simulink library "LookupModeling"  (Simulink 7.7)
settings: Solver=ode45  StartTime=0.0  StopTime=10.0  RelTol=1e-3
settings Model: Creator=medcps  LastModifiedBy=iris

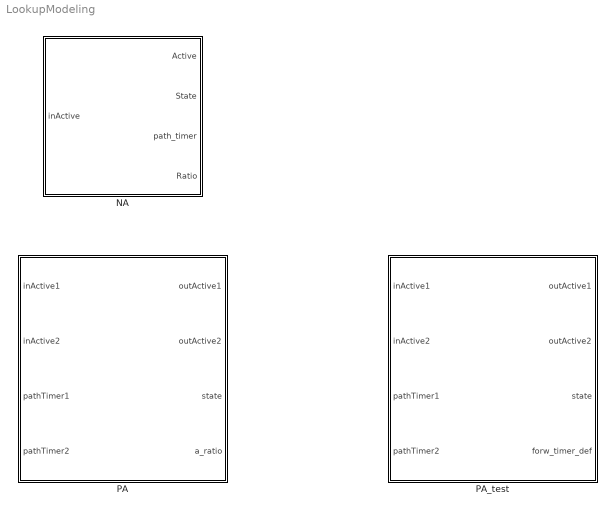
== system LookupModeling ==
  NA : Subsystem  mask{TERP_s_m=100, TERP_defs_m=100, TRRP_s_m=100, TRRP_def_m=100, Trest_s_m=100, Trest_def_m=100, Terp_min_m=100, Terp_max_m=100}
      mask prompts: TERP_s_m "Terp Start"; TERP_defs_m "Terp Default Start"; TRRP_s_m "Trrp Start"; TRRP_def_m "Trrp Default"; Trest_s_m "Trest Start"; Trest_def_m "Trest Default"; Terp_min_m "Terp Min"; Terp_max_m "Terp Max"
  PA : Subsystem  mask{min_path_par_m=0, bck_param_m=0, forw_param_m=0, a_ratio_table_m=0}
      mask prompts: min_path_par_m "Min Path Param"; bck_param_m "Back Param"; forw_param_m "Fwd Param"; a_ratio_table_m "Ratio Table Source"
  PA_test : Subsystem  mask{min_path_par_m=0, bck_param_m=0, forw_param_m=0}
      mask prompts: min_path_par_m "Min Path Param"; bck_param_m "Back Param"; forw_param_m "Fwd Param"

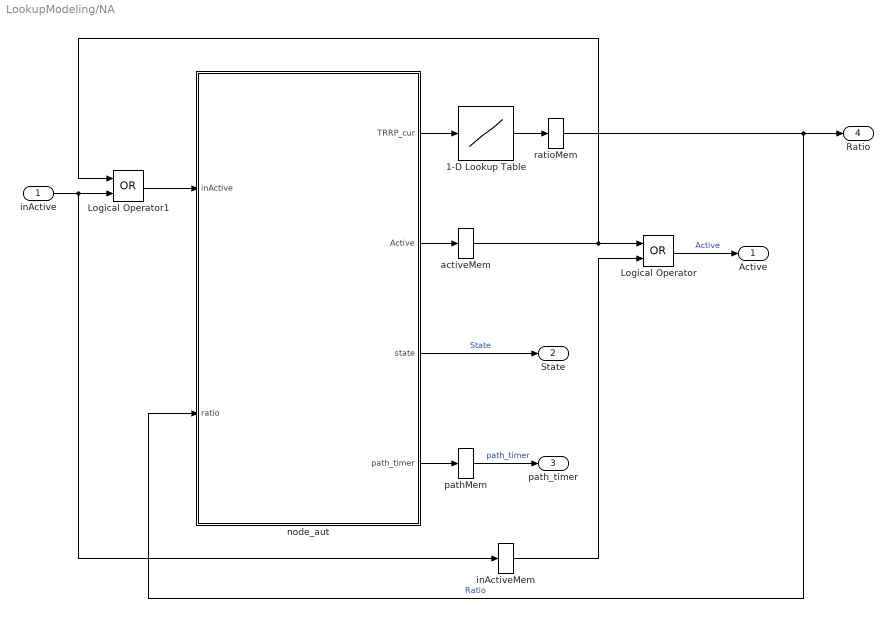
== system LookupModeling/NA ==
  inActive : Inport
  1-D Lookup Table : Lookup_n-D  NumberOfTableDimensions=1  BreakpointsForDimension1=[0:TRRP_def_m]  IndexSearchMethod=Evenly spaced points  Table=[0:1/TRRP_def_m:1]  InterpMethod=Flat  ExtrapMethod=Clip  DiagnosticForOutOfRangeInput=Error  UseLastTableValue=on  OutMin=0  OutMax=1  OutDataTypeStr=fixdt(0,8,7)  RndMeth=Zero  InputSameDT=on
  Logical Operator : Logic  Operator=OR  AllPortsSameDT=off  OutDataTypeStr=boolean
  Logical Operator1 : Logic  Operator=OR  AllPortsSameDT=off  OutDataTypeStr=boolean
  activeMem : Memory  InheritSampleTime=on
  inActiveMem : Memory  InheritSampleTime=on
  node_aut : Stateflow chart  TreatAsAtomicUnit=on
  pathMem : Memory  InheritSampleTime=on
  ratioMem : Memory  InheritSampleTime=on
  Active : Outport
  State : Outport  Port=2
  path_timer : Outport  Port=3
  Ratio : Outport  Port=4  OutMin=0  OutMax=1  OutDataTypeStr=fixdt(0,8,7)  LockScale=on
  wires:
  pathMem/1 -> path_timer/1  "path_timer"
  Logical Operator/1 -> Active/1  "Active"
  inActiveMem/1 -> Logical Operator/2
  Logical Operator1/1 -> node_aut/1(inActive)
  inActive/1 -> inActiveMem/1, Logical Operator1/2
  activeMem/1 -> Logical Operator/1, Logical Operator1/1
  ratioMem/1 -> Ratio/1, node_aut/2(ratio)  "Ratio"
  node_aut/1(TRRP_cur) -> 1-D Lookup Table/1
  1-D Lookup Table/1 -> ratioMem/1
  node_aut/2(Active) -> activeMem/1
  node_aut/3(state) -> State/1  "State"
  node_aut/4(path_timer) -> pathMem/1

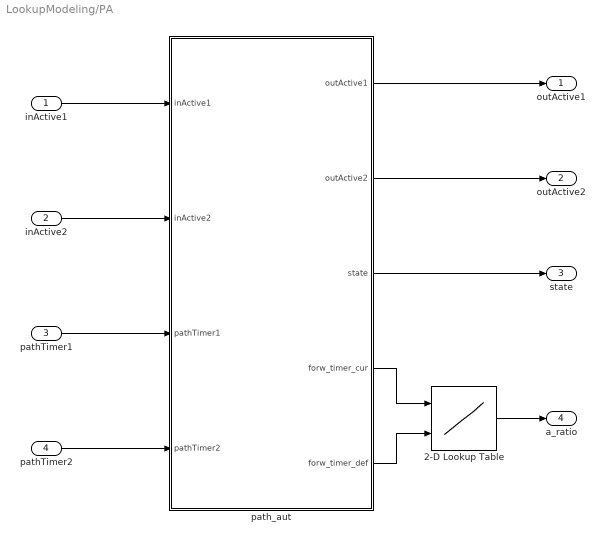
== system LookupModeling/PA ==
  inActive1 : Inport
  inActive2 : Inport  Port=2
  pathTimer1 : Inport  Port=3
  pathTimer2 : Inport  Port=4
  2-D Lookup Table : Lookup_n-D  BreakpointsForDimension1=[0:forw_param_m*3]  BreakpointsForDimension2=[0:forw_param_m*3]  IndexSearchMethod=Evenly spaced points  Table=a_ratio_table_m  TableDataTypeStr=fixdt(0,16,14)  InterpMethod=Flat  DiagnosticForOutOfRangeInput=Error  OutDataTypeStr=fixdt(0,16,14)  RndMeth=Simplest  InputSameDT=on  LockScale=on
  path_aut : Stateflow chart  TreatAsAtomicUnit=on
  outActive1 : Outport
  outActive2 : Outport  Port=2
  state : Outport  Port=3
  a_ratio : Outport  Port=4  OutDataTypeStr=fixdt(0,16,14)
  wires:
  inActive2/1 -> path_aut/2(inActive2)
  inActive1/1 -> path_aut/1(inActive1)
  pathTimer1/1 -> path_aut/3(pathTimer1)
  pathTimer2/1 -> path_aut/4(pathTimer2)
  path_aut/1(outActive1) -> outActive1/1
  path_aut/2(outActive2) -> outActive2/1
  path_aut/3(state) -> state/1
  path_aut/4(forw_timer_cur) -> 2-D Lookup Table/1
  path_aut/5(forw_timer_def) -> 2-D Lookup Table/2
  2-D Lookup Table/1 -> a_ratio/1

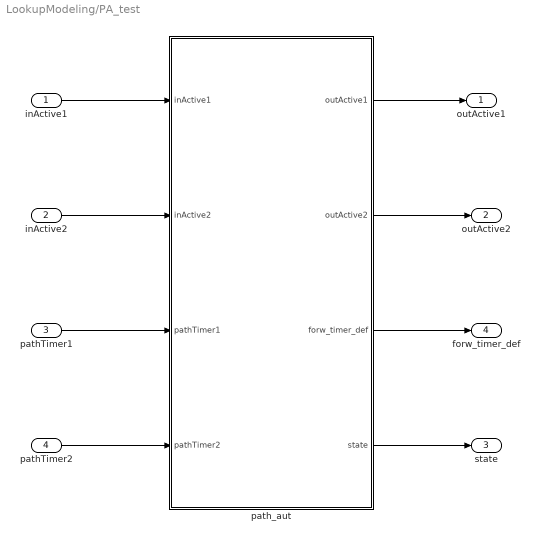
== system LookupModeling/PA_test ==
  inActive1 : Inport
  inActive2 : Inport  Port=2
  pathTimer1 : Inport  Port=3
  pathTimer2 : Inport  Port=4
  path_aut : Stateflow chart  TreatAsAtomicUnit=on
  outActive1 : Outport
  outActive2 : Outport  Port=2
  state : Outport  Port=3
  forw_timer_def : Outport  Port=4
  wires:
  path_aut/4(state) -> state/1
  path_aut/2(outActive2) -> outActive2/1
  path_aut/1(outActive1) -> outActive1/1
  pathTimer2/1 -> path_aut/4(pathTimer2)
  pathTimer1/1 -> path_aut/3(pathTimer1)
  inActive1/1 -> path_aut/1(inActive1)
  inActive2/1 -> path_aut/2(inActive2)
  path_aut/3(forw_timer_def) -> forw_timer_def/1

== stateflow chart NA/node_aut ==
  settings: executeAtInitialization=1
  state NodeAutomaton
    state Rest
      du: Trest_cur = Trest_cur-1;
      du: state=1;
    state RRP
      du: TRRP_cur = TRRP_cur-1;
      du: state=3;
    state ERP
      ex: Active = 0;
      du: TERP_cur = TERP_cur-1;
      du: path_timer = 0;
      du: Active = 0;
      du: state=2;
    (default) -> Rest : {Active=0;
        | Trest_cur = Trest_s;TERP_def=TERP_defs;
        | TERP_cur = TERP_s;
        | TRRP_cur = TRRP_s;
        | path_timer = 0;}
    Rest -> ERP [order 2] : [inActive]
        | {Trest_cur = Trest_def;
        | TERP_def = Terp_max;
        | TERP_cur = Terp_max;
        | path_timer = 1;}
    ERP -> ERP [order 1] : [inActive]
        | {TERP_cur = Terp_min;
        | TERP_def = Terp_min;
        | path_timer = 3;}
    RRP -> ERP [order 1] : [inActive]
        | {
        | TERP_def = Terp_min + ((Terp_max-Terp_min)* (1C-ratio)*(1C-ratio)*(1C-ratio));
        | path_timer = 1+2*ratio*ratio;
        | TERP_cur = TERP_def;
        | TRRP_cur = TRRP_def;
        | }
    Rest -> ERP [order 1] : [(~inActive) & (Trest_cur==0)]
        | {Trest_cur = Trest_def;
        | Active = 1;
        | path_timer = 0;}
    ERP -> RRP [order 2] : [(~inActive) & (TERP_cur==0)]
        | {TERP_cur = TERP_def;
        | path_timer = 0;}
    RRP -> Rest [order 2] : [(~inActive) & (TRRP_cur==0)]
        | {TRRP_cur = TRRP_def;
        | path_timer = 0;}
  data: TERP_cur local uint16; TRRP_cur output uint16; Trest_cur local uint16; TERP_defs constant uint16 =TERP_defs_m; TRRP_def constant uint16 =TRRP_def_m; Trest_def constant uint16 =Trest_def_m; Active output boolean; inActive input boolean; TERP_s constant uint16 =TERP_s_m; TRRP_s constant uint16 =TRRP_s_m; Trest_s constant uint16 =Trest_s_m; Terp_min constant uint16 =Terp_min_m; Terp_max constant uint16 =Terp_max_m; TERP_def local uint16; state output uint8; path_timer output fixdt(0,16,14) [0..3]; ratio input fixdt(0,8,7) [0..1]

== stateflow chart PA_test/path_aut ==
  settings: executeAtInitialization=1
  state PathAutomaton [parallel]
    settings: executionOrder=3
    state Idle
      en: idle_st = 1;
      du: state=1;
    state AntegradeConduction
      du: forw_timer_cur = forw_timer_cur-1;
      du: outActive1=0;
      du: idle_st = 0;
      du: state=2;
    state Double
      du: forw_timer_cur = forw_timer_cur-1;
      du: bck_timer_cur = bck_timer_cur-1;
      du: state=5;
    state RetrogradeConduction
      du: bck_timer_cur = bck_timer_cur-1;
      du: outActive2=0;
      du: state=3;
    state Conflict
      ex: outActive2=0;
      ex: outActive1=0;
      du: state=4;
    (default) -> Idle : {outActive1=0;
        | outActive2=0;}
    Idle -> AntegradeConduction [order 1] : [inActive1]
    Idle -> RetrogradeConduction [order 2] : [(~inActive1)&&(inActive2)]
    AntegradeConduction -> Double [order 1] : [inActive2]
    Conflict -> Idle
    AntegradeConduction -> Conflict [order 2] : [forw_timer_cur==0 && (~inActive2)]
        | {forw_timer_cur=forw_timer_def;
        | outActive2=1;}
    RetrogradeConduction -> Double [order 2] : [inActive1]
    RetrogradeConduction -> Conflict [order 1] : [bck_timer_cur==0 && (~inActive1)]
        | {bck_timer_cur=bck_timer_def;
        | outActive1=1;}
    Double -> AntegradeConduction [order 1] : [bck_timer_cur==0]
        | {bck_timer_cur=bck_timer_def;
        | outActive1=1;}
    Double -> RetrogradeConduction [order 3] : [forw_timer_cur==0]
        | {forw_timer_cur=forw_timer_def;
        | outActive2=1;}
    Double -> Conflict [order 2] : [(forw_timer_cur != 0) && (bck_timer_cur != 0)]
        | {forw_timer_cur=forw_timer_def;
        | bck_timer_cur=bck_timer_def;}
  state UpdateForward [parallel]
    settings: executionOrder=1
    state Update
    UpdateForward.Update -> UpdateForward.Update [order 1] : [(pathTimer1 > 0) && (idle_st)]
        | {forw_timer_def = forw_param * pathTimer1;
        |  forw_timer_cur = forw_timer_def;}
    UpdateForward.Update -> UpdateForward.Update [order 2] : [(pathTimer1 > 0) && (~idle_st)]
        | {forw_timer_def = forw_param * pathTimer1;}
  state UpdateBackward [parallel]
    settings: executionOrder=2
    state Update
    UpdateBackward.Update -> UpdateBackward.Update [order 1] : [(pathTimer2 > 0) && (idle_st)]
        | {bck_timer_def = bck_param * pathTimer2;
        |  bck_timer_cur = bck_timer_def;}
    UpdateBackward.Update -> UpdateBackward.Update [order 2] : [(pathTimer2 > 0) && (~idle_st)]
        | {bck_timer_def = bck_param * pathTimer2;}
  data: forw_timer_cur local uint16; bck_timer_cur local uint16; outActive1 output boolean; inActive1 input boolean; inActive2 input boolean; outActive2 output boolean; min_path_par constant uint16 =min_path_par_m; bck_timer_def local uint16; forw_timer_def output uint16; bck_param constant uint16 =bck_param_m; forw_param constant uint16 =forw_param_m; idle_st local boolean; state output uint8; pathTimer1 input fixdt(0,16,14) [0..3]; pathTimer2 input fixdt(0,16,14) [0..3]

== stateflow chart PA/path_aut ==
  settings: executeAtInitialization=1
  state PathAutomaton [parallel]
    settings: executionOrder=3
    state Idle
      en: idle_st = 1;
      du: state=1;
    state AntegradeConduction
      du: forw_timer_cur = forw_timer_cur-1;
      du: outActive1=0;
      du: idle_st = 0;
      du: state=2;
    state Double
      du: forw_timer_cur = forw_timer_cur-1;
      du: bck_timer_cur = bck_timer_cur-1;
      du: state=5;
    state RetrogradeConduction
      du: bck_timer_cur = bck_timer_cur-1;
      du: outActive2=0;
      du: state=3;
    state Conflict
      ex: outActive2=0;
      ex: outActive1=0;
      du: state=4;
    (default) -> Idle : {outActive1=0;
        | outActive2=0;}
    Idle -> AntegradeConduction [order 1] : [inActive1]
    Idle -> RetrogradeConduction [order 2] : [(~inActive1)&&(inActive2)]
    AntegradeConduction -> Double [order 1] : [inActive2]
    Conflict -> Idle
    AntegradeConduction -> Conflict [order 2] : [forw_timer_cur==0 && (~inActive2)]
        | {forw_timer_cur=forw_timer_def;
        | outActive2=1;}
    RetrogradeConduction -> Double [order 2] : [inActive1]
    RetrogradeConduction -> Conflict [order 1] : [bck_timer_cur==0 && (~inActive1)]
        | {bck_timer_cur=bck_timer_def;
        | outActive1=1;}
    Double -> AntegradeConduction [order 1] : [bck_timer_cur==0]
        | {bck_timer_cur=bck_timer_def;
        | outActive1=1;}
    Double -> RetrogradeConduction [order 3] : [forw_timer_cur==0]
        | {forw_timer_cur=forw_timer_def;
        | outActive2=1;}
    Double -> Conflict [order 2] : [(forw_timer_cur != 0) && (bck_timer_cur != 0)]
        | {forw_timer_cur=forw_timer_def;
        | bck_timer_cur=bck_timer_def;}
  state UpdateForward [parallel]
    settings: executionOrder=1
    state Update
    UpdateForward.Update -> UpdateForward.Update [order 1] : [(pathTimer1 > 0) && (idle_st)]
        | {forw_timer_def = forw_param * pathTimer1;
        |  forw_timer_cur = forw_timer_def;}
    UpdateForward.Update -> UpdateForward.Update [order 2] : [(pathTimer1 > 0) && (~idle_st)]
        | {forw_timer_def = forw_param * pathTimer1;}
  state UpdateBackward [parallel]
    settings: executionOrder=2
    state Update
    UpdateBackward.Update -> UpdateBackward.Update [order 1] : [(pathTimer2 > 0) && (idle_st)]
        | {bck_timer_def = bck_param * pathTimer2;
        |  bck_timer_cur = bck_timer_def;}
    UpdateBackward.Update -> UpdateBackward.Update [order 2] : [(pathTimer2 > 0) && (~idle_st)]
        | {bck_timer_def = bck_param * pathTimer2;}
  data: bck_timer_cur local uint16; outActive1 output boolean; inActive1 input boolean; inActive2 input boolean; outActive2 output boolean; min_path_par constant uint16 =min_path_par_m; bck_timer_def local uint16; bck_param constant uint16 =bck_param_m; forw_param constant uint16 =forw_param_m; idle_st local boolean; state output uint8; forw_timer_cur output uint16; forw_timer_def output uint16; pathTimer1 input fixdt(0,16,14) [0..3]; pathTimer2 input fixdt(0,16,14) [0..3]
